simulink model "Figure2"  (R2025b)
settings: Solver=VariableStepAuto  StartTime=0.0  StopTime=10.0  RelTol=1e-3
values from neighbouring files (symbols this model uses):
  P1 = A*7    (= 77)    [Attempt.m]
  P2 = B*800    (= 8000)    [Attempt.m]
  P3 = C*8    (= 80)    [Attempt.m]
  P4 = D*700    (= 11900)    [Attempt.m]
  P5 = E*600    (= 10800)    [Attempt.m]
  P6 = F*50    (= 500)    [Attempt.m]
  P7 = G*500    (= 6000)    [Attempt.m]
  P8 = H*5    (= 50)    [Attempt.m]
settings Model: Creator=hashaamzafar  LastModifiedBy=hashaamzafar

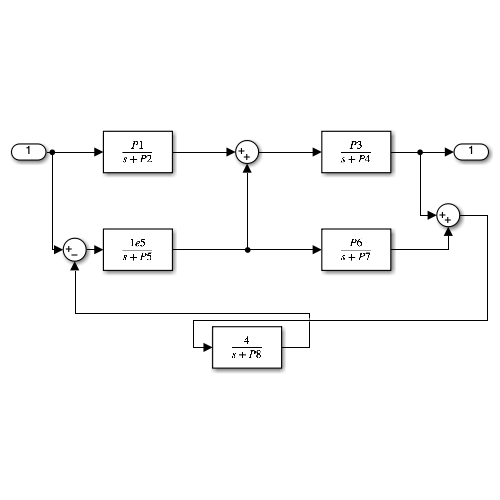
[thumbnail: Simulink's stored preview of the top-level diagram]
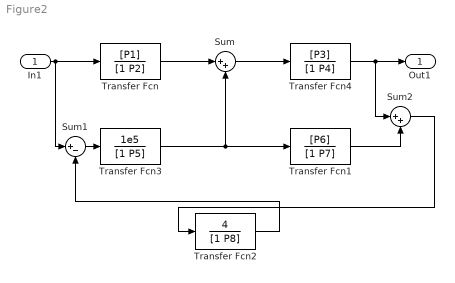
== system Figure2 ==
  In1 : Inport
  Sum : Sum  Inputs=|++
  Sum1 : Sum  Inputs=|+-
  Sum2 : Sum  Inputs=|++
  Transfer Fcn : TransferFcn  Numerator=[P1]  Denominator=[1 P2]
  Transfer Fcn1 : TransferFcn  Numerator=[P6]  Denominator=[1 P7]
  Transfer Fcn2 : TransferFcn  Numerator=[4]  Denominator=[1 P8]
  Transfer Fcn3 : TransferFcn  Numerator=[1e5]  Denominator=[1 P5]
  Transfer Fcn4 : TransferFcn  Numerator=[P3]  Denominator=[1 P4]
  Out1 : Outport
  wires:
  In1/1 -> Sum1/1, Transfer Fcn/1
  Transfer Fcn/1 -> Sum/1
  Sum1/1 -> Transfer Fcn3/1
  Sum/1 -> Transfer Fcn4/1
  Transfer Fcn4/1 -> Out1/1, Sum2/1
  Transfer Fcn3/1 -> Transfer Fcn1/1, Sum/2
  Transfer Fcn2/1 -> Sum1/2
  Transfer Fcn1/1 -> Sum2/2
  Sum2/1 -> Transfer Fcn2/1
